simulink model "hyd_hyb_2_int_cont_Final_AMT"  (R2013b)
settings: Solver=ode4  StartTime=0  StopTime=3005  FixedStep=0.01  MaxStep=.4  RelTol=1e-8
InitFcn:
  | const_3_new
values from neighbouring files (symbols this model uses):
  Af = 6.3    [brk_enrg.m]    (also in brk_enrg_1.m)
  BSFC_906_205 = [3.5684 4.3466 5.1668 6.0769 6.988 7.8992 8.8104 9.7336 10.8548 11.9809 13.1112 14.2571 ... (663 elements, 39x17)]    [BSFC_map_906_205.mat]
  Cd = 0.55    [brk_enrg.m]    (also in brk_enrg_1.m)
  den = 1.202    [brk_enrg.m]    (also in brk_enrg_1.m)
  fr = 0.01    [brk_enrg.m]    (also in brk_enrg_1.m)
undefined symbols (not defined in the file or in its folder): clutchRise, down_spd_2, down_spd_3, down_spd_4, down_spd_c, Driving_Cycle, fuel_density, gearshift, I_wheel, Idle_spd_eng_906, M1_hydr, p_v_15, pmax_125, qv_125, Rw, sec_eng_sfc_map, T0, T1, T_max_906, T_min, TC_spd_ratio_max, teta_new_10, torque_convertor, Twait, up_spd_1, up_spd_2, up_spd_3, up_spd_c, v_p_10, v_p_15, v_p_5
libraries: neural x1742, fl_lib x43, nesl_utility x30, sdl_lib x14, simulink x4, simulink_need_slupdate x1
(part 18 of 26)

== system hyd_hyb_2_int_cont_Final_AMT/controller1/optimized controller/SOC upper 0.5/SOC upper 0.6/SOC under 0.7/net_loc_rod_6_7/Layer 3/Delays 1 ==
  "p{3}" : Inport  PortDimensions=65
  mux : Mux  Inputs=1
  "pd{3,2}" : Outport
  wires:
  mux/1 -> "pd{3,2}"/1
  "p{3}"/1 -> mux/1

== system hyd_hyb_2_int_cont_Final_AMT/controller1/optimized controller/SOC upper 0.5/SOC upper 0.6/SOC under 0.7/net_loc_rod_6_7/Layer 3/LW{3,2} ==
  "ad{3,2}" : Inport  PortDimensions=65
  "IW{3,2}(1,:)'" : Constant  Value=[-0.21190558148273514;-0.028250456332647261;0.33957139945877679;0.19274652478953275;-0.42961698454965908;0.23052255270038227;-0.37497561736022994;-0.06185645589928139;0.01165116263494341;-0.15963912751743919;-0.87324175537425064;0.10590816804656823;0.069053323215663556;0.077910861425516578;-0.16798922620742043;-0.22056720645742031;0.13367494956427081;0.36136249854843466;-0.50239119110845365;0.012331807086952057;-0.096965686807043844;0.11986982112408856;-0.31830050450261449;0.11706810526331732;-0.52980599528072625;-0.29641942316489694;0.17415062016965829;-0.098905843864114676;-0.27508713459790696;-0.033419612327731621;-0.2254339214197735;0.027831220456353004;0.29925289926941745;-0.070435212430303012;0.29619502791901131;-0.47601606724683371;-0.22767027734105019;0.41339738030579964;-0.26217552491145868;-0.036734014287553567;-0.55981845033730226;-0.83512658858317002;-0.056808057570803309;-0.22345195834484222;-0.28036785465301478;-0.22949243361228511;-0.34209162741874338;-0.39092697900045326;0.32531105678992528;0.10423076111174255;0.2359871210092597;-0.47216686128522006;-0.20439924920680128;-0.11922663531256097;-0.019922601561886109;0.044510324605291363;-0.27729290371229609;-0.36614438332522081;0.816368987577891;0.54191447654746938;0.5157713773005137;0.26230341773617905;0.70532547287095315;0.23331847514630705;-0.046156806107243299]
  Mux : Mux  Inputs=1
  dotprod1 : neural/Weight Functions/dotprod
  "lz{3,2}" : Outport
  wires:
  Mux/1 -> "lz{3,2}"/1
  dotprod1/1 -> Mux/1
  "ad{3,2}"/1 -> dotprod1/2
  "IW{3,2}(1,:)'"/1 -> dotprod1/1

== system hyd_hyb_2_int_cont_Final_AMT/controller1/optimized controller/SOC upper 0.5/SOC upper 0.6/SOC upper 0.7/SOC under 0.8/net_col_a_b_7_8/Layer 1 ==
  "p{1}" : Inport  PortDimensions=2
  Delays 1 : Subsystem
  "IW{1,1}" : Subsystem
  "b{1}" : Constant  Value=[8.2916467646585872;-7.8114778185757023;-7.3358740319827671;-6.8287428687854348;6.3257902864971145;5.7992770695782818;5.3094756346830199;4.9115066356687667;-4.3713108462153514;-3.8883509962050646;3.3793456803311566;2.8729633399532961;-2.4756245359899856;1.6763370386535841;1.5305900525159519;0.90882364470135646;0.44992343591511891;0.040547487289665569;0.62387277578531353;-1.1506418258106572;1.8779212144940651;1.9372314274500504;2.3477899083139837;2.9384613260166579;-3.1569713919719704;3.945195331065702;-4.46999394454709;-4.8935944330051546;5.3383406441107919;-5.8921601467554003;-6.437017113135763;-6.6308369147221251;-7.2519979683223239;7.7912717207669244;-8.2765880656885411]
  netsum : Sum  Inputs=2  SaturateOnIntegerOverflow=on  InputSameDT=on  OutDataTypeStr=Inherit: Same as first input
  tansig : neural/Transfer Functions/tansig
  "a{1}" : Outport  InitialOutput=[0;0;0;0;0;0;0;0;0;0;0;0;0;0;0;0;0;0;0;0;0;0;0;0;0;0;0;0;0;0;0;0;0;0;0]
  wires:
  tansig/1 -> "a{1}"/1
  netsum/1 -> tansig/1
  "b{1}"/1 -> netsum/2
  "IW{1,1}"/1("iz{1,1}") -> netsum/1
  Delays 1/1("pd{1,1}") -> "IW{1,1}"/1("pd{1,1}")
  "p{1}"/1 -> Delays 1/1("p{1}")

== system hyd_hyb_2_int_cont_Final_AMT/controller1/optimized controller/SOC upper 0.5/SOC upper 0.6/SOC upper 0.7/SOC under 0.8/net_col_a_b_7_8/Layer 2 ==
  "a{1} " : Inport  PortDimensions=35
  Delays 1 : Subsystem
  "LW{2,1}" : Subsystem
  "b{2}" : Constant  Value=[1.6246025903810972;-1.5137529513143568;1.4133649641113548;1.3507873768326613;1.2831264026044094;-1.1583875849183927;-1.1687705629463485;-1.0638601573162123;-0.97507485546902606;-0.92163063226781328;-0.85414749875120755;-0.81745251898413263;0.71780688605314269;0.64596911275152968;-0.5713050323286234;0.44864531658767243;-0.44458366605836119;-0.39178178454963697;-0.30831552725782874;-0.2030923610966566;-0.17177709670230834;-0.089970322460785082;0.045878470178160817;0.077082912036474494;-0.18386481774142041;0.2395566239489996;0.27679632832356704;0.35435254107540132;0.43035932518500436;-0.49005207867104572;-0.61109910818045332;-0.69212605142728045;-0.70628312057121345;0.72592925676845665;-0.82226073192444138;-0.92563474243113997;0.91244556659384735;1.0573029525194646;1.1239522443373839;1.2068081707832854;1.2709694444207866;1.357007844557339;-1.4138174953273674;1.4928009886700373;1.5432286468653338]
  netsum : Sum  Inputs=2  SaturateOnIntegerOverflow=on  InputSameDT=on  OutDataTypeStr=Inherit: Same as first input
  tansig : neural/Transfer Functions/tansig
  "a{2}" : Outport  InitialOutput=[0;0;0;0;0;0;0;0;0;0;0;0;0;0;0;0;0;0;0;0;0;0;0;0;0;0;0;0;0;0;0;0;0;0;0;0;0;0;0;0;0;0;0;0;0]
  wires:
  tansig/1 -> "a{2}"/1
  netsum/1 -> tansig/1
  "b{2}"/1 -> netsum/2
  "LW{2,1}"/1("lz{2,1}") -> netsum/1
  Delays 1/1("pd{2,1}") -> "LW{2,1}"/1("ad{2,1}")
  "a{1} "/1 -> Delays 1/1("p{2}")

== system hyd_hyb_2_int_cont_Final_AMT/controller1/optimized controller/SOC upper 0.5/SOC upper 0.6/SOC upper 0.7/SOC under 0.8/net_col_a_b_7_8/Layer 3 ==
  "a{2} " : Inport  PortDimensions=45
  Delays 1 : Subsystem
  "LW{3,2}" : Subsystem
  "b{3}" : Constant  Value=0.43583087047788488
  netsum : Sum  Inputs=2  SaturateOnIntegerOverflow=on  InputSameDT=on  OutDataTypeStr=Inherit: Same as first input
  purelin : neural/Transfer Functions/purelin
  "a{3}" : Outport  InitialOutput=0
  wires:
  purelin/1 -> "a{3}"/1
  netsum/1 -> purelin/1
  "b{3}"/1 -> netsum/2
  "LW{3,2}"/1("lz{3,2}") -> netsum/1
  Delays 1/1("pd{3,2}") -> "LW{3,2}"/1("ad{3,2}")
  "a{2} "/1 -> Delays 1/1("p{3}")

== system hyd_hyb_2_int_cont_Final_AMT/controller1/optimized controller/SOC upper 0.5/SOC upper 0.6/SOC upper 0.7/SOC under 0.8/net_col_a_b_7_8/Process Input 1 ==
  x : Inport  PortDimensions=2
  fixunknowns : neural/Processing Functions/fixunknowns  inputSize=2  indices=[1 2]
  mapminmax : neural/Processing Functions/mapminmax  xmin=[0.0050576114402896234;0.2341095]  xmax=[1;0.94609200000000004]  ymin=-1  ymax=1
  removeconstantrows : neural/Processing Functions/removeconstantrows  inputSize=2  keep=[1 2]
  p : Outport  PortDimensions=2
  wires:
  mapminmax/1 -> p/1
  removeconstantrows/1 -> mapminmax/1
  fixunknowns/1 -> removeconstantrows/1
  x/1 -> fixunknowns/1

== system hyd_hyb_2_int_cont_Final_AMT/controller1/optimized controller/SOC upper 0.5/SOC upper 0.6/SOC upper 0.7/SOC under 0.8/net_col_a_b_7_8/Process Output 1 ==
  a : Inport  PortDimensions=1
  mapminmax_reverse : neural/Processing Functions/mapminmax_reverse  xmin=0  xmax=1  ymin=-1  ymax=1
  removeconstantrows_reverse : neural/Processing Functions/removeconstantrows_reverse  inputSize=1  constants=zeros(0,1)  rearrange=1
  y : Outport  PortDimensions=1
  wires:
  removeconstantrows_reverse/1 -> y/1
  mapminmax_reverse/1 -> removeconstantrows_reverse/1
  a/1 -> mapminmax_reverse/1

== system hyd_hyb_2_int_cont_Final_AMT/controller1/optimized controller/SOC upper 0.5/SOC upper 0.6/SOC upper 0.7/SOC under 0.8/net_col_c_d_7_8/Layer 1 ==
  "p{1}" : Inport  PortDimensions=2
  Delays 1 : Subsystem
  "IW{1,1}" : Subsystem
  "b{1}" : Constant  Value=[8.3116902859191448;7.8029060171194731;7.2867035561831317;6.8260213470550735;6.346607988807234;5.8562497365900965;-5.3743261762591725;4.9530955883541345;-4.383911258273109;-3.8970793742576069;-3.4314686513161763;2.863791263998738;2.4209773053043331;1.956446882392439;-1.4732357207624023;-0.86517942611961574;-0.48032492618428974;-0.026719041791466704;0.45434793064694279;0.96417086831869769;-1.4746840868110174;-1.932288244085119;-2.4708323565900367;-2.9643399257520366;-3.430878366683491;3.8862801103928728;4.3962114473631928;4.8870263091686326;-5.3420629575502314;-5.8367411293877227;-6.4407592729025556;6.809228192120738;7.3082174034078067;7.795329331848893;8.3148626555089304]
  netsum : Sum  Inputs=2  SaturateOnIntegerOverflow=on  InputSameDT=on  OutDataTypeStr=Inherit: Same as first input
  tansig : neural/Transfer Functions/tansig
  "a{1}" : Outport  InitialOutput=[0;0;0;0;0;0;0;0;0;0;0;0;0;0;0;0;0;0;0;0;0;0;0;0;0;0;0;0;0;0;0;0;0;0;0]
  wires:
  tansig/1 -> "a{1}"/1
  netsum/1 -> tansig/1
  "b{1}"/1 -> netsum/2
  "IW{1,1}"/1("iz{1,1}") -> netsum/1
  Delays 1/1("pd{1,1}") -> "IW{1,1}"/1("pd{1,1}")
  "p{1}"/1 -> Delays 1/1("p{1}")

== system hyd_hyb_2_int_cont_Final_AMT/controller1/optimized controller/SOC upper 0.5/SOC upper 0.6/SOC upper 0.7/SOC under 0.8/net_col_c_d_7_8/Layer 2 ==
  "a{1} " : Inport  PortDimensions=35
  Delays 1 : Subsystem
  "LW{2,1}" : Subsystem
  "b{2}" : Constant  Value=[-1.5686018942941038;-1.4913194182180465;1.4364195261274875;1.3923653246708561;-1.3174444073080744;-1.2329202605406324;-1.2231091177906401;-1.1113434209070936;1.0523981087233136;-1.0082372091808669;-0.93678500720920321;-0.85933642747852601;0.79256290609693925;0.7194191061208759;0.62735773675601636;-0.63057612726771706;0.52881759345176838;0.4726739238819378;-0.36991235182195747;0.39954692502574662;0.32402525688235295;-0.25368530430266362;-0.16353113859080878;0.1147228728047736;-0.058400493998987592;0.033005568957060874;-0.052329484615956483;-0.10924330494808851;-0.19798005180984199;-0.29896342389825387;0.35766529096251598;0.42867990671694767;0.4489209967696316;0.53972993122561663;0.6167646902802062;-0.61139064819023359;-0.74306982939588972;-0.76508190452300739;-0.87147423129092416;0.94153999709968716;-0.99016236737475172;-1.0232275653663527;-1.1417743437718129;1.1612439923201026;-1.1779260494401698;1.2812899302236036;1.3707661966465723;1.4742421981136882;-1.47793500374455;-1.5586030678282377]
  netsum : Sum  Inputs=2  SaturateOnIntegerOverflow=on  InputSameDT=on  OutDataTypeStr=Inherit: Same as first input
  tansig : neural/Transfer Functions/tansig
  "a{2}" : Outport  InitialOutput=[0;0;0;0;0;0;0;0;0;0;0;0;0;0;0;0;0;0;0;0;0;0;0;0;0;0;0;0;0;0;0;0;0;0;0;0;0;0;0;0;0;0;0;0;0;0;0;0;0;0]
  wires:
  tansig/1 -> "a{2}"/1
  netsum/1 -> tansig/1
  "b{2}"/1 -> netsum/2
  "LW{2,1}"/1("lz{2,1}") -> netsum/1
  Delays 1/1("pd{2,1}") -> "LW{2,1}"/1("ad{2,1}")
  "a{1} "/1 -> Delays 1/1("p{2}")

== system hyd_hyb_2_int_cont_Final_AMT/controller1/optimized controller/SOC upper 0.5/SOC upper 0.6/SOC upper 0.7/SOC under 0.8/net_col_c_d_7_8/Layer 3 ==
  "a{2} " : Inport  PortDimensions=50
  Delays 1 : Subsystem
  "LW{3,2}" : Subsystem
  "b{3}" : Constant  Value=-0.33436314693187646
  netsum : Sum  Inputs=2  SaturateOnIntegerOverflow=on  InputSameDT=on  OutDataTypeStr=Inherit: Same as first input
  purelin : neural/Transfer Functions/purelin
  "a{3}" : Outport  InitialOutput=0
  wires:
  purelin/1 -> "a{3}"/1
  netsum/1 -> purelin/1
  "b{3}"/1 -> netsum/2
  "LW{3,2}"/1("lz{3,2}") -> netsum/1
  Delays 1/1("pd{3,2}") -> "LW{3,2}"/1("ad{3,2}")
  "a{2} "/1 -> Delays 1/1("p{3}")

== system hyd_hyb_2_int_cont_Final_AMT/controller1/optimized controller/SOC upper 0.5/SOC upper 0.6/SOC upper 0.7/SOC under 0.8/net_col_c_d_7_8/Process Input 1 ==
  x : Inport  PortDimensions=2
  fixunknowns : neural/Processing Functions/fixunknowns  inputSize=2  indices=[1 2]
  mapminmax : neural/Processing Functions/mapminmax  xmin=[0.11115622208057092;0.17457650000000002]  xmax=[1;0.653254]  ymin=-1  ymax=1
  removeconstantrows : neural/Processing Functions/removeconstantrows  inputSize=2  keep=[1 2]
  p : Outport  PortDimensions=2
  wires:
  mapminmax/1 -> p/1
  removeconstantrows/1 -> mapminmax/1
  fixunknowns/1 -> removeconstantrows/1
  x/1 -> fixunknowns/1

== system hyd_hyb_2_int_cont_Final_AMT/controller1/optimized controller/SOC upper 0.5/SOC upper 0.6/SOC upper 0.7/SOC under 0.8/net_col_c_d_7_8/Process Output 1 ==
  a : Inport  PortDimensions=1
  mapminmax_reverse : neural/Processing Functions/mapminmax_reverse  xmin=0  xmax=1  ymin=-1  ymax=1
  removeconstantrows_reverse : neural/Processing Functions/removeconstantrows_reverse  inputSize=1  constants=zeros(0,1)  rearrange=1
  y : Outport  PortDimensions=1
  wires:
  removeconstantrows_reverse/1 -> y/1
  mapminmax_reverse/1 -> removeconstantrows_reverse/1
  a/1 -> mapminmax_reverse/1

== system hyd_hyb_2_int_cont_Final_AMT/controller1/optimized controller/SOC upper 0.5/SOC upper 0.6/SOC upper 0.7/SOC under 0.8/net_col_e_f_7_8/Layer 1 ==
  "p{1}" : Inport  PortDimensions=2
  Delays 1 : Subsystem
  "IW{1,1}" : Subsystem
  "b{1}" : Constant  Value=[-7.6881018002993811;-7.1696124955463407;6.6274067676391244;-6.1028538948157074;-5.5114890432277486;5.0228105143392874;-4.3713949897040196;-3.9579533195973844;-3.5424320446653481;-2.9063109252236838;2.3884921851729382;-1.8701611263712352;-1.3278082575057837;-0.7034153508496056;-0.29496096693313423;-0.24905479630949848;0.64349556452967571;-1.3288485356492385;-1.8412347415254877;2.3729253819088352;2.9176813905058485;-3.4852070547888778;-3.9696003266601889;-4.4547493683646611;-5.0158733055263856;5.560382862684909;6.0845307363798815;-6.6092525461039449;7.1485320918848041;7.6474074439409838]
  netsum : Sum  Inputs=2  SaturateOnIntegerOverflow=on  InputSameDT=on  OutDataTypeStr=Inherit: Same as first input
  tansig : neural/Transfer Functions/tansig
  "a{1}" : Outport  InitialOutput=[0;0;0;0;0;0;0;0;0;0;0;0;0;0;0;0;0;0;0;0;0;0;0;0;0;0;0;0;0;0]
  wires:
  tansig/1 -> "a{1}"/1
  netsum/1 -> tansig/1
  "b{1}"/1 -> netsum/2
  "IW{1,1}"/1("iz{1,1}") -> netsum/1
  Delays 1/1("pd{1,1}") -> "IW{1,1}"/1("pd{1,1}")
  "p{1}"/1 -> Delays 1/1("p{1}")

== system hyd_hyb_2_int_cont_Final_AMT/controller1/optimized controller/SOC upper 0.5/SOC upper 0.6/SOC upper 0.7/SOC under 0.8/net_col_e_f_7_8/Layer 2 ==
  "a{1} " : Inport  PortDimensions=30
  Delays 1 : Subsystem
  "LW{2,1}" : Subsystem
  "b{2}" : Constant  Value=[-1.5477297612963636;-1.5293021250108161;-1.4865534978599506;-1.4350225305745659;-1.3320349172545887;1.2759493127119488;1.2067092228755465;1.1585040165641989;1.0818111732552;-1.0217707490071199;-0.93625284533737974;0.86084334590742473;-0.81611566901033294;-0.75977572837522622;-0.68195671405109437;0.61250166315132237;0.56784720520380716;-0.47392917471101453;-0.42294051348806871;-0.34059086854467668;0.28432035961595142;-0.26239849492555123;0.16655305034653378;0.09689078681840467;-0.043301963584861977;0.032103319387171828;0.13394593375940797;0.18086752211467982;-0.1880786349548369;-0.29610569226816436;0.35856623667981335;-0.44696828544509076;0.48850426202371683;-0.4992446928319636;0.60332468246739523;-0.68407090563130457;0.75073264123508454;0.83254585737929787;0.85952336377303395;-0.95829921584290212;1.0048957119927975;1.0901091238963656;-1.1625782212970923;1.206521081803045;1.2660766711955194;-1.3373607373409551;-1.4184409448334543;1.4527994853647119;1.5068978308092387;1.6095996810907955]
  netsum : Sum  Inputs=2  SaturateOnIntegerOverflow=on  InputSameDT=on  OutDataTypeStr=Inherit: Same as first input
  tansig : neural/Transfer Functions/tansig
  "a{2}" : Outport  InitialOutput=[0;0;0;0;0;0;0;0;0;0;0;0;0;0;0;0;0;0;0;0;0;0;0;0;0;0;0;0;0;0;0;0;0;0;0;0;0;0;0;0;0;0;0;0;0;0;0;0;0;0]
  wires:
  tansig/1 -> "a{2}"/1
  netsum/1 -> tansig/1
  "b{2}"/1 -> netsum/2
  "LW{2,1}"/1("lz{2,1}") -> netsum/1
  Delays 1/1("pd{2,1}") -> "LW{2,1}"/1("ad{2,1}")
  "a{1} "/1 -> Delays 1/1("p{2}")

== system hyd_hyb_2_int_cont_Final_AMT/controller1/optimized controller/SOC upper 0.5/SOC upper 0.6/SOC upper 0.7/SOC under 0.8/net_col_e_f_7_8/Layer 3 ==
  "a{2} " : Inport  PortDimensions=50
  Delays 1 : Subsystem
  "LW{3,2}" : Subsystem
  "b{3}" : Constant  Value=-0.46106071391077463
  netsum : Sum  Inputs=2  SaturateOnIntegerOverflow=on  InputSameDT=on  OutDataTypeStr=Inherit: Same as first input
  purelin : neural/Transfer Functions/purelin
  "a{3}" : Outport  InitialOutput=0
  wires:
  purelin/1 -> "a{3}"/1
  netsum/1 -> purelin/1
  "b{3}"/1 -> netsum/2
  "LW{3,2}"/1("lz{3,2}") -> netsum/1
  Delays 1/1("pd{3,2}") -> "LW{3,2}"/1("ad{3,2}")
  "a{2} "/1 -> Delays 1/1("p{3}")

== system hyd_hyb_2_int_cont_Final_AMT/controller1/optimized controller/SOC upper 0.5/SOC upper 0.6/SOC upper 0.7/SOC under 0.8/net_col_e_f_7_8/Process Input 1 ==
  x : Inport  PortDimensions=2
  fixunknowns : neural/Processing Functions/fixunknowns  inputSize=2  indices=[1 2]
  mapminmax : neural/Processing Functions/mapminmax  xmin=[0.00010433375339546994;0.0080852249999999997]  xmax=[1.009090909090909;0.64359999999999995]  ymin=-1  ymax=1
  removeconstantrows : neural/Processing Functions/removeconstantrows  inputSize=2  keep=[1 2]
  p : Outport  PortDimensions=2
  wires:
  mapminmax/1 -> p/1
  removeconstantrows/1 -> mapminmax/1
  fixunknowns/1 -> removeconstantrows/1
  x/1 -> fixunknowns/1

== system hyd_hyb_2_int_cont_Final_AMT/controller1/optimized controller/SOC upper 0.5/SOC upper 0.6/SOC upper 0.7/SOC under 0.8/net_col_e_f_7_8/Process Output 1 ==
  a : Inport  PortDimensions=1
  mapminmax_reverse : neural/Processing Functions/mapminmax_reverse  xmin=0  xmax=1  ymin=-1  ymax=1
  removeconstantrows_reverse : neural/Processing Functions/removeconstantrows_reverse  inputSize=1  constants=zeros(0,1)  rearrange=1
  y : Outport  PortDimensions=1
  wires:
  removeconstantrows_reverse/1 -> y/1
  mapminmax_reverse/1 -> removeconstantrows_reverse/1
  a/1 -> mapminmax_reverse/1

== system hyd_hyb_2_int_cont_Final_AMT/controller1/optimized controller/SOC upper 0.5/SOC upper 0.6/SOC upper 0.7/SOC under 0.8/net_loc_rod_7_8/Layer 1 ==
  "p{1}" : Inport  PortDimensions=2
  Delays 1 : Subsystem
  "IW{1,1}" : Subsystem
  "b{1}" : Constant  Value=[-7.6664348708937533;7.1445971682878477;6.6167168492832911;6.0860061370357288;-5.5315107878025573;5.0261307682562233;-4.494082622797607;4.0719078555663542;3.4709759431734448;2.9188468639647454;2.3943935266761707;1.8335702310625019;1.3202491244505703;-0.76888435535120259;0.24778438862887789;0.33462371266191271;-0.76243416083955973;1.3762346449687806;1.9102702785135495;-2.3929428850095324;-2.9022803344286112;-3.690412197637341;3.9573609372276932;-4.5993292631946163;-5.0475261103641618;5.4709604300797592;6.077408482873671;6.5770239742392009;7.1375905348778197;7.6179993162728579]
  netsum : Sum  Inputs=2  SaturateOnIntegerOverflow=on  InputSameDT=on  OutDataTypeStr=Inherit: Same as first input
  tansig : neural/Transfer Functions/tansig
  "a{1}" : Outport  InitialOutput=[0;0;0;0;0;0;0;0;0;0;0;0;0;0;0;0;0;0;0;0;0;0;0;0;0;0;0;0;0;0]
  wires:
  tansig/1 -> "a{1}"/1
  netsum/1 -> tansig/1
  "b{1}"/1 -> netsum/2
  "IW{1,1}"/1("iz{1,1}") -> netsum/1
  Delays 1/1("pd{1,1}") -> "IW{1,1}"/1("pd{1,1}")
  "p{1}"/1 -> Delays 1/1("p{1}")

== system hyd_hyb_2_int_cont_Final_AMT/controller1/optimized controller/SOC upper 0.5/SOC upper 0.6/SOC upper 0.7/SOC under 0.8/net_loc_rod_7_8/Layer 2 ==
  "a{1} " : Inport  PortDimensions=30
  Delays 1 : Subsystem
  "LW{2,1}" : Subsystem
  "b{2}" : Constant  Value=[1.5809057638664712;1.5807151854123314;1.4855560118917412;1.4342816648463235;-1.3852838862690111;-1.3763643250737478;-1.2699307671350113;1.2284424739443496;-1.1667825506616738;1.1126454079697519;1.0473054037992569;0.99287875006871451;-0.95329260687326012;0.83638794087360679;-0.83792818135557123;-0.78046148241162161;-0.71425010683179146;0.68949490542424974;0.64329890641382304;0.57899988405152292;-0.47143091913162039;-0.47926974452184956;-0.40398687055644222;-0.35659194048479592;0.30321322377409698;-0.27451350524017853;-0.1767238128948169;0.16987849996636148;0.080295435290659523;-0.029950542574714353;0.027089350482413167;0.058629507356316252;0.15615280386139965;-0.20370835576685978;0.24221681438327167;0.28202876584714487;-0.38246747542268622;0.41676300939491745;-0.45528940316231631;0.52075351132689529;-0.571489263720799;0.64385068877791618;-0.69328786198464676;0.7382904151092311;-0.7686738347751072;0.84397313956728726;-0.88866651589897194;0.96837105796755452;1.0162563106498559;-1.0533618556353999;-1.0943063056832119;-1.1877806527843298;-1.2159917192725045;-1.253506527704173;1.3326748437569171;1.3938223174811426;1.4658688434887885;1.4916223339098742;1.5398710502961235;1.601176272795612]
  netsum : Sum  Inputs=2  SaturateOnIntegerOverflow=on  InputSameDT=on  OutDataTypeStr=Inherit: Same as first input
  tansig : neural/Transfer Functions/tansig
  "a{2}" : Outport  InitialOutput=[0;0;0;0;0;0;0;0;0;0;0;0;0;0;0;0;0;0;0;0;0;0;0;0;0;0;0;0;0;0;0;0;0;0;0;0;0;0;0;0;0;0;0;0;0;0;0;0;0;0;0;0;0;0;0;0;0;0;0;0]
  wires:
  tansig/1 -> "a{2}"/1
  netsum/1 -> tansig/1
  "b{2}"/1 -> netsum/2
  "LW{2,1}"/1("lz{2,1}") -> netsum/1
  Delays 1/1("pd{2,1}") -> "LW{2,1}"/1("ad{2,1}")
  "a{1} "/1 -> Delays 1/1("p{2}")

== system hyd_hyb_2_int_cont_Final_AMT/controller1/optimized controller/SOC upper 0.5/SOC upper 0.6/SOC upper 0.7/SOC under 0.8/net_loc_rod_7_8/Layer 3 ==
  "a{2} " : Inport  PortDimensions=60
  Delays 1 : Subsystem
  "LW{3,2}" : Subsystem
  "b{3}" : Constant  Value=-0.93224771825496566
  netsum : Sum  Inputs=2  SaturateOnIntegerOverflow=on  InputSameDT=on  OutDataTypeStr=Inherit: Same as first input
  purelin : neural/Transfer Functions/purelin
  "a{3}" : Outport  InitialOutput=0
  wires:
  purelin/1 -> "a{3}"/1
  netsum/1 -> purelin/1
  "b{3}"/1 -> netsum/2
  "LW{3,2}"/1("lz{3,2}") -> netsum/1
  Delays 1/1("pd{3,2}") -> "LW{3,2}"/1("ad{3,2}")
  "a{2} "/1 -> Delays 1/1("p{3}")

== system hyd_hyb_2_int_cont_Final_AMT/controller1/optimized controller/SOC upper 0.5/SOC upper 0.6/SOC upper 0.7/SOC under 0.8/net_loc_rod_7_8/Process Input 1 ==
  x : Inport  PortDimensions=2
  fixunknowns : neural/Processing Functions/fixunknowns  inputSize=2  indices=[1 2]
  mapminmax : neural/Processing Functions/mapminmax  xmin=[0.088429741348767466;0.013660410000000001]  xmax=[1;0.49235399999999996]  ymin=-1  ymax=1
  removeconstantrows : neural/Processing Functions/removeconstantrows  inputSize=2  keep=[1 2]
  p : Outport  PortDimensions=2
  wires:
  mapminmax/1 -> p/1
  removeconstantrows/1 -> mapminmax/1
  fixunknowns/1 -> removeconstantrows/1
  x/1 -> fixunknowns/1

== system hyd_hyb_2_int_cont_Final_AMT/controller1/optimized controller/SOC upper 0.5/SOC upper 0.6/SOC upper 0.7/SOC under 0.8/net_loc_rod_7_8/Process Output 1 ==
  a : Inport  PortDimensions=1
  mapminmax_reverse : neural/Processing Functions/mapminmax_reverse  xmin=0  xmax=1  ymin=-1  ymax=1
  removeconstantrows_reverse : neural/Processing Functions/removeconstantrows_reverse  inputSize=1  constants=zeros(0,1)  rearrange=1
  y : Outport  PortDimensions=1
  wires:
  removeconstantrows_reverse/1 -> y/1
  mapminmax_reverse/1 -> removeconstantrows_reverse/1
  a/1 -> mapminmax_reverse/1

== system hyd_hyb_2_int_cont_Final_AMT/controller1/optimized controller/SOC upper 0.5/SOC upper 0.6/SOC upper 0.7/SOC upper 0.8/net_col_a_b_8_9/Layer 1 ==
  "p{1}" : Inport  PortDimensions=2
  Delays 1 : Subsystem
  "IW{1,1}" : Subsystem
  "b{1}" : Constant  Value=[8.2903358215080676;-7.7657998848495637;7.3258361320457999;6.8322940827755767;6.3907366524362228;5.8513299473215454;5.428748873413956;4.8908030844795327;4.4622980602266207;3.9184323697946635;3.4421533237276636;-2.8848117854051845;-2.3908374697190853;1.9426308888625365;-1.4634502352179708;1.0159704232714091;-0.47136167422531949;-0.025928304818340971;0.48223344450605304;0.95348009234162501;1.5262155812589833;-1.9494027462808818;-2.378648219600497;-2.9433743702973341;3.2998478685400348;-3.8872063221167878;4.433440918095731;-4.8693917332986398;5.3487774127091638;5.8086420838160704;-6.3275200720026099;-6.8387453294921219;7.3072846143090002;7.798095465885619;8.2978794542543266]
  netsum : Sum  Inputs=2  SaturateOnIntegerOverflow=on  InputSameDT=on  OutDataTypeStr=Inherit: Same as first input
  tansig : neural/Transfer Functions/tansig
  "a{1}" : Outport  InitialOutput=[0;0;0;0;0;0;0;0;0;0;0;0;0;0;0;0;0;0;0;0;0;0;0;0;0;0;0;0;0;0;0;0;0;0;0]
  wires:
  tansig/1 -> "a{1}"/1
  netsum/1 -> tansig/1
  "b{1}"/1 -> netsum/2
  "IW{1,1}"/1("iz{1,1}") -> netsum/1
  Delays 1/1("pd{1,1}") -> "IW{1,1}"/1("pd{1,1}")
  "p{1}"/1 -> Delays 1/1("p{1}")

== system hyd_hyb_2_int_cont_Final_AMT/controller1/optimized controller/SOC upper 0.5/SOC upper 0.6/SOC upper 0.7/SOC upper 0.8/net_col_a_b_8_9/Layer 2 ==
  "a{1} " : Inport  PortDimensions=35
  Delays 1 : Subsystem
  "LW{2,1}" : Subsystem
  "b{2}" : Constant  Value=[1.5516475171408779;1.4835098818771537;1.4312277511141751;-1.3698842963986313;-1.2806997344309183;-1.1693837969306802;-1.1407058875630671;-1.0781990386589757;-1.0357595176145418;0.90372054013783332;0.85261985678638907;0.76193934695339194;0.75173184958776618;0.66413214424768063;0.5671249522564511;0.51661208652598578;0.40848110978741226;0.36021562083255332;-0.28984413185003965;-0.21008240837066611;-0.10811356805866763;0.078212987099658043;0.050261178409190178;-0.062855911586719854;-0.15960669841975192;-0.29221472137958321;0.30888189547496875;-0.37759084863654085;0.39785437443106902;0.5025042997703113;0.6852123648390992;0.57126476826852779;-0.72454872028325679;-0.81256808327758079;0.92122536494791152;-0.94207467763840702;1.0352444398307015;1.0564038748070703;1.1414641552110378;1.1803996896086595;-1.3183578069980528;-1.3096087100254543;1.3521491510226666;1.5210842316929682;1.5661396273710371]
  netsum : Sum  Inputs=2  SaturateOnIntegerOverflow=on  InputSameDT=on  OutDataTypeStr=Inherit: Same as first input
  tansig : neural/Transfer Functions/tansig
  "a{2}" : Outport  InitialOutput=[0;0;0;0;0;0;0;0;0;0;0;0;0;0;0;0;0;0;0;0;0;0;0;0;0;0;0;0;0;0;0;0;0;0;0;0;0;0;0;0;0;0;0;0;0]
  wires:
  tansig/1 -> "a{2}"/1
  netsum/1 -> tansig/1
  "b{2}"/1 -> netsum/2
  "LW{2,1}"/1("lz{2,1}") -> netsum/1
  Delays 1/1("pd{2,1}") -> "LW{2,1}"/1("ad{2,1}")
  "a{1} "/1 -> Delays 1/1("p{2}")

== system hyd_hyb_2_int_cont_Final_AMT/controller1/optimized controller/SOC upper 0.5/SOC upper 0.6/SOC upper 0.7/SOC upper 0.8/net_col_a_b_8_9/Layer 3 ==
  "a{2} " : Inport  PortDimensions=45
  Delays 1 : Subsystem
  "LW{3,2}" : Subsystem
  "b{3}" : Constant  Value=0.6155887857634984
  netsum : Sum  Inputs=2  SaturateOnIntegerOverflow=on  InputSameDT=on  OutDataTypeStr=Inherit: Same as first input
  purelin : neural/Transfer Functions/purelin
  "a{3}" : Outport  InitialOutput=0
  wires:
  purelin/1 -> "a{3}"/1
  netsum/1 -> purelin/1
  "b{3}"/1 -> netsum/2
  "LW{3,2}"/1("lz{3,2}") -> netsum/1
  Delays 1/1("pd{3,2}") -> "LW{3,2}"/1("ad{3,2}")
  "a{2} "/1 -> Delays 1/1("p{3}")

== system hyd_hyb_2_int_cont_Final_AMT/controller1/optimized controller/SOC upper 0.5/SOC upper 0.6/SOC upper 0.7/SOC upper 0.8/net_col_a_b_8_9/Process Input 1 ==
  x : Inport  PortDimensions=2
  fixunknowns : neural/Processing Functions/fixunknowns  inputSize=2  indices=[1 2]
  mapminmax : neural/Processing Functions/mapminmax  xmin=[0.0003822621604903857;0.041431750000000003]  xmax=[1;0.69701880000000005]  ymin=-1  ymax=1
  removeconstantrows : neural/Processing Functions/removeconstantrows  inputSize=2  keep=[1 2]
  p : Outport  PortDimensions=2
  wires:
  mapminmax/1 -> p/1
  removeconstantrows/1 -> mapminmax/1
  fixunknowns/1 -> removeconstantrows/1
  x/1 -> fixunknowns/1

== system hyd_hyb_2_int_cont_Final_AMT/controller1/optimized controller/SOC upper 0.5/SOC upper 0.6/SOC upper 0.7/SOC upper 0.8/net_col_a_b_8_9/Process Output 1 ==
  a : Inport  PortDimensions=1
  mapminmax_reverse : neural/Processing Functions/mapminmax_reverse  xmin=0  xmax=1  ymin=-1  ymax=1
  removeconstantrows_reverse : neural/Processing Functions/removeconstantrows_reverse  inputSize=1  constants=zeros(0,1)  rearrange=1
  y : Outport  PortDimensions=1
  wires:
  removeconstantrows_reverse/1 -> y/1
  mapminmax_reverse/1 -> removeconstantrows_reverse/1
  a/1 -> mapminmax_reverse/1

== system hyd_hyb_2_int_cont_Final_AMT/controller1/optimized controller/SOC upper 0.5/SOC upper 0.6/SOC upper 0.7/SOC upper 0.8/net_col_c_d_8_9/Layer 1 ==
  "p{1}" : Inport  PortDimensions=2
  Delays 1 : Subsystem
  "IW{1,1}" : Subsystem
  "b{1}" : Constant  Value=[-7.6524589954305595;7.1575966111085725;-6.654801813906313;-6.062921949452706;-5.5671598839301657;-5.0521178951183314;4.5110838179576307;3.946782880463152;3.4022759889300365;-2.9332570607530637;2.3847485055726749;1.930372285371202;-1.4382019821303194;0.77000183863714244;-0.26225474692650153;-0.20738493161860463;0.79875786224452561;1.314952811728606;1.8171463545761435;2.2799587853155048;2.9303600998292048;3.4808110827958494;3.9748206575799894;4.5187216997884914;-5.0721055404459179;5.5382016443803641;6.2740684597329439;6.4514085496008367;-7.3392600553068776;7.5659178060488959]
  netsum : Sum  Inputs=2  SaturateOnIntegerOverflow=on  InputSameDT=on  OutDataTypeStr=Inherit: Same as first input
  tansig : neural/Transfer Functions/tansig
  "a{1}" : Outport  InitialOutput=[0;0;0;0;0;0;0;0;0;0;0;0;0;0;0;0;0;0;0;0;0;0;0;0;0;0;0;0;0;0]
  wires:
  tansig/1 -> "a{1}"/1
  netsum/1 -> tansig/1
  "b{1}"/1 -> netsum/2
  "IW{1,1}"/1("iz{1,1}") -> netsum/1
  Delays 1/1("pd{1,1}") -> "IW{1,1}"/1("pd{1,1}")
  "p{1}"/1 -> Delays 1/1("p{1}")

== system hyd_hyb_2_int_cont_Final_AMT/controller1/optimized controller/SOC upper 0.5/SOC upper 0.6/SOC upper 0.7/SOC upper 0.8/net_col_c_d_8_9/Layer 2 ==
  "a{1} " : Inport  PortDimensions=30
  Delays 1 : Subsystem
  "LW{2,1}" : Subsystem
  "b{2}" : Constant  Value=[-1.5287022483014878;1.5426403940657185;-1.4614221356586912;1.3400868618459401;-1.2027676831476171;-1.2178358987324378;-1.0910327499881933;-1.0404872041228237;-0.9206407025162644;0.82096842682832016;-0.81597475436367373;0.70513330671674967;0.5942273025863497;-0.57573907549896008;-0.36643092989287496;-0.41499221347877618;0.27330592040460605;-0.19900672217238721;0.12188682845735625;0.099377692896292932;-0.048454168804516924;0.11918352171058183;-0.2007677246837809;-0.26479653336079806;-0.34453332666848635;0.42671542704119692;0.5146335294347133;0.62751706753897618;-0.67658170183233923;-0.79975832025806681;-0.86684211752692231;-0.92593317836401323;1.0152616108508217;1.0935118102424268;-1.184870758657562;-1.2348820260904967;1.3200273808778371;1.4157163141339153;-1.4512197794490678;1.574504628514257]
  netsum : Sum  Inputs=2  SaturateOnIntegerOverflow=on  InputSameDT=on  OutDataTypeStr=Inherit: Same as first input
  tansig : neural/Transfer Functions/tansig
  "a{2}" : Outport  InitialOutput=[0;0;0;0;0;0;0;0;0;0;0;0;0;0;0;0;0;0;0;0;0;0;0;0;0;0;0;0;0;0;0;0;0;0;0;0;0;0;0;0]
  wires:
  tansig/1 -> "a{2}"/1
  netsum/1 -> tansig/1
  "b{2}"/1 -> netsum/2
  "LW{2,1}"/1("lz{2,1}") -> netsum/1
  Delays 1/1("pd{2,1}") -> "LW{2,1}"/1("ad{2,1}")
  "a{1} "/1 -> Delays 1/1("p{2}")

== system hyd_hyb_2_int_cont_Final_AMT/controller1/optimized controller/SOC upper 0.5/SOC upper 0.6/SOC upper 0.7/SOC upper 0.8/net_col_c_d_8_9/Layer 3 ==
  "a{2} " : Inport  PortDimensions=40
  Delays 1 : Subsystem
  "LW{3,2}" : Subsystem
  "b{3}" : Constant  Value=0.9979622803312711
  netsum : Sum  Inputs=2  SaturateOnIntegerOverflow=on  InputSameDT=on  OutDataTypeStr=Inherit: Same as first input
  purelin : neural/Transfer Functions/purelin
  "a{3}" : Outport  InitialOutput=0
  wires:
  purelin/1 -> "a{3}"/1
  netsum/1 -> purelin/1
  "b{3}"/1 -> netsum/2
  "LW{3,2}"/1("lz{3,2}") -> netsum/1
  Delays 1/1("pd{3,2}") -> "LW{3,2}"/1("ad{3,2}")
  "a{2} "/1 -> Delays 1/1("p{3}")

== system hyd_hyb_2_int_cont_Final_AMT/controller1/optimized controller/SOC upper 0.5/SOC upper 0.6/SOC upper 0.7/SOC upper 0.8/net_col_c_d_8_9/Process Input 1 ==
  x : Inport  PortDimensions=2
  fixunknowns : neural/Processing Functions/fixunknowns  inputSize=2  indices=[1 2]
  mapminmax : neural/Processing Functions/mapminmax  xmin=[0.0094276106161651479;0.0091891777777777812]  xmax=[1;0.58245800000000003]  ymin=-1  ymax=1
  removeconstantrows : neural/Processing Functions/removeconstantrows  inputSize=2  keep=[1 2]
  p : Outport  PortDimensions=2
  wires:
  mapminmax/1 -> p/1
  removeconstantrows/1 -> mapminmax/1
  fixunknowns/1 -> removeconstantrows/1
  x/1 -> fixunknowns/1

== system hyd_hyb_2_int_cont_Final_AMT/controller1/optimized controller/SOC upper 0.5/SOC upper 0.6/SOC upper 0.7/SOC upper 0.8/net_col_c_d_8_9/Process Output 1 ==
  a : Inport  PortDimensions=1
  mapminmax_reverse : neural/Processing Functions/mapminmax_reverse  xmin=0  xmax=1  ymin=-1  ymax=1
  removeconstantrows_reverse : neural/Processing Functions/removeconstantrows_reverse  inputSize=1  constants=zeros(0,1)  rearrange=1
  y : Outport  PortDimensions=1
  wires:
  removeconstantrows_reverse/1 -> y/1
  mapminmax_reverse/1 -> removeconstantrows_reverse/1
  a/1 -> mapminmax_reverse/1

== system hyd_hyb_2_int_cont_Final_AMT/controller1/optimized controller/SOC upper 0.5/SOC upper 0.6/SOC upper 0.7/SOC upper 0.8/net_col_e_f_8_9/Layer 1 ==
  "p{1}" : Inport  PortDimensions=2
  Delays 1 : Subsystem
  "IW{1,1}" : Subsystem
  "b{1}" : Constant  Value=[9.4015860759943966;-8.9623532948495601;8.5480536519185701;8.1046505410424192;-7.5466355394940079;-7.2605592645199044;-6.7644609711250361;-6.40324068377633;6.0469685190620748;-5.7413104529964567;5.1004073550828455;4.7536909688907976;-4.3869298322884216;-3.7118385502056612;3.4173879876904838;-2.9642792238956539;2.5109440040112929;2.1436189865847459;-1.7054760294924085;1.2789285491357323;0.84702857546792387;-0.42845582688182682;0.054882353957567492;-0.40580987731936785;0.83189682774366758;-1.3323426667166121;1.7017266340694932;2.2140395237166892;-2.4800599409674757;2.8411443376504515;-3.3611018732833946;-3.9122774496765476;-4.2725122406999256;4.2536055601757869;5.1225152835425725;-5.5373788998665079;5.9765064965422576;-6.4270271409881659;-6.791830750517736;-7.3042677014218906;-7.6961747552868962;8.0679800328071796;-8.5403581573270912;-8.9645856768191319;9.3914854194720938]
  netsum : Sum  Inputs=2  SaturateOnIntegerOverflow=on  InputSameDT=on  OutDataTypeStr=Inherit: Same as first input
  tansig : neural/Transfer Functions/tansig
  "a{1}" : Outport  InitialOutput=[0;0;0;0;0;0;0;0;0;0;0;0;0;0;0;0;0;0;0;0;0;0;0;0;0;0;0;0;0;0;0;0;0;0;0;0;0;0;0;0;0;0;0;0;0]
  wires:
  tansig/1 -> "a{1}"/1
  netsum/1 -> tansig/1
  "b{1}"/1 -> netsum/2
  "IW{1,1}"/1("iz{1,1}") -> netsum/1
  Delays 1/1("pd{1,1}") -> "IW{1,1}"/1("pd{1,1}")
  "p{1}"/1 -> Delays 1/1("p{1}")

== system hyd_hyb_2_int_cont_Final_AMT/controller1/optimized controller/SOC upper 0.5/SOC upper 0.6/SOC upper 0.7/SOC upper 0.8/net_col_e_f_8_9/Layer 2 ==
  "a{1} " : Inport  PortDimensions=45
  Delays 1 : Subsystem
  "LW{2,1}" : Subsystem
  "b{2}" : Constant  Value=[1.5253321238047128;1.4426726863252606;-1.3964076148505893;-1.3434292293770562;1.2678530519528122;1.1669163880968327;-1.1241349942514887;-1.0917726034495538;-1.0179705297074282;-0.95676753272242343;0.880004094253938;0.82779411887496857;0.77361446766304676;-0.70961133316188985;0.67547417475024096;0.59353382732856175;0.52119438118217298;0.42939358344025758;-0.40583901134992156;-0.33670536350227231;-0.30812213039158887;0.21614184544915765;-0.15827865619741779;0.052978289767213006;-0.0318222212966148;0.030995499762107467;0.089872985526170221;0.170835823291382;-0.23422224909781603;0.3147508551030011;-0.39562127859636015;0.4016708983328201;-0.46047284059491694;-0.51954829349618004;0.58569212638724233;0.65270315684131097;-0.67454354069254074;0.80243169197463704;0.85133965435293057;0.8963147932673079;-0.96395548478725546;-1.0113939551973554;1.108860035215596;1.084747261067099;1.2150548435091166;-1.2765324018453701;-1.3515968421724327;-1.3804162913221047;1.4444549438943957;1.5249712838830871]
  netsum : Sum  Inputs=2  SaturateOnIntegerOverflow=on  InputSameDT=on  OutDataTypeStr=Inherit: Same as first input
  tansig : neural/Transfer Functions/tansig
  "a{2}" : Outport  InitialOutput=[0;0;0;0;0;0;0;0;0;0;0;0;0;0;0;0;0;0;0;0;0;0;0;0;0;0;0;0;0;0;0;0;0;0;0;0;0;0;0;0;0;0;0;0;0;0;0;0;0;0]
  wires:
  tansig/1 -> "a{2}"/1
  netsum/1 -> tansig/1
  "b{2}"/1 -> netsum/2
  "LW{2,1}"/1("lz{2,1}") -> netsum/1
  Delays 1/1("pd{2,1}") -> "LW{2,1}"/1("ad{2,1}")
  "a{1} "/1 -> Delays 1/1("p{2}")

== system hyd_hyb_2_int_cont_Final_AMT/controller1/optimized controller/SOC upper 0.5/SOC upper 0.6/SOC upper 0.7/SOC upper 0.8/net_col_e_f_8_9/Layer 3 ==
  "a{2} " : Inport  PortDimensions=50
  Delays 1 : Subsystem
  "LW{3,2}" : Subsystem
  "b{3}" : Constant  Value=-0.73453859105110131
  netsum : Sum  Inputs=2  SaturateOnIntegerOverflow=on  InputSameDT=on  OutDataTypeStr=Inherit: Same as first input
  purelin : neural/Transfer Functions/purelin
  "a{3}" : Outport  InitialOutput=0
  wires:
  purelin/1 -> "a{3}"/1
  netsum/1 -> purelin/1
  "b{3}"/1 -> netsum/2
  "LW{3,2}"/1("lz{3,2}") -> netsum/1
  Delays 1/1("pd{3,2}") -> "LW{3,2}"/1("ad{3,2}")
  "a{2} "/1 -> Delays 1/1("p{3}")

== system hyd_hyb_2_int_cont_Final_AMT/controller1/optimized controller/SOC upper 0.5/SOC upper 0.6/SOC upper 0.7/SOC upper 0.8/net_col_e_f_8_9/Process Input 1 ==
  x : Inport  PortDimensions=2
  fixunknowns : neural/Processing Functions/fixunknowns  inputSize=2  indices=[1 2]
  mapminmax : neural/Processing Functions/mapminmax  xmin=[0.012187384778861551;0.026488162500000002]  xmax=[1.009090909090909;0.54223299999999997]  ymin=-1  ymax=1
  removeconstantrows : neural/Processing Functions/removeconstantrows  inputSize=2  keep=[1 2]
  p : Outport  PortDimensions=2
  wires:
  mapminmax/1 -> p/1
  removeconstantrows/1 -> mapminmax/1
  fixunknowns/1 -> removeconstantrows/1
  x/1 -> fixunknowns/1

== system hyd_hyb_2_int_cont_Final_AMT/controller1/optimized controller/SOC upper 0.5/SOC upper 0.6/SOC upper 0.7/SOC upper 0.8/net_col_e_f_8_9/Process Output 1 ==
  a : Inport  PortDimensions=1
  mapminmax_reverse : neural/Processing Functions/mapminmax_reverse  xmin=0  xmax=1  ymin=-1  ymax=1
  removeconstantrows_reverse : neural/Processing Functions/removeconstantrows_reverse  inputSize=1  constants=zeros(0,1)  rearrange=1
  y : Outport  PortDimensions=1
  wires:
  removeconstantrows_reverse/1 -> y/1
  mapminmax_reverse/1 -> removeconstantrows_reverse/1
  a/1 -> mapminmax_reverse/1

== system hyd_hyb_2_int_cont_Final_AMT/controller1/optimized controller/SOC upper 0.5/SOC upper 0.6/SOC upper 0.7/SOC upper 0.8/net_loc_rod_8_9/Layer 1 ==
  "p{1}" : Inport  PortDimensions=2
  Delays 1 : Subsystem
  "IW{1,1}" : Subsystem
  "b{1}" : Constant  Value=[6.9957007495819052;-6.4222898500365853;-5.788068254476527;4.9484038597923208;-4.897680334949869;4.0902305007500548;-3.4579527463580804;-2.7707675590821905;2.2287546877108686;-1.770011467044045;-1.1837111909482061;-0.033766395640138086;-0.010074994472143614;-0.76903616379233108;1.1855446863873538;1.7401032750561261;2.4956626318889397;2.9273420606852465;-3.5487048822941847;-3.9918574108068756;-4.3619449722476942;5.2498961119747447;-5.6249161050042025;6.4634990534294996;6.9541097039616186]
  netsum : Sum  Inputs=2  SaturateOnIntegerOverflow=on  InputSameDT=on  OutDataTypeStr=Inherit: Same as first input
  tansig : neural/Transfer Functions/tansig
  "a{1}" : Outport  InitialOutput=[0;0;0;0;0;0;0;0;0;0;0;0;0;0;0;0;0;0;0;0;0;0;0;0;0]
  wires:
  tansig/1 -> "a{1}"/1
  netsum/1 -> tansig/1
  "b{1}"/1 -> netsum/2
  "IW{1,1}"/1("iz{1,1}") -> netsum/1
  Delays 1/1("pd{1,1}") -> "IW{1,1}"/1("pd{1,1}")
  "p{1}"/1 -> Delays 1/1("p{1}")

== system hyd_hyb_2_int_cont_Final_AMT/controller1/optimized controller/SOC upper 0.5/SOC upper 0.6/SOC upper 0.7/SOC upper 0.8/net_loc_rod_8_9/Layer 2 ==
  "a{1} " : Inport  PortDimensions=25
  Delays 1 : Subsystem
  "LW{2,1}" : Subsystem
  "b{2}" : Constant  Value=[3.285738559317775;-3.0376074370088557;2.9182454057119536;2.7178352616345638;-2.4587927074579339;-2.4627649650599852;2.3023381037248565;2.1198885946639727;1.8964367137641158;-1.753810639868139;-1.6118339248574409;1.3623437270724821;1.2373583426900003;-1.0632509377280692;-0.90198498135918437;0.67954961164333982;-0.5916625396957329;0.40151715963968393;-0.23710697987107432;-0.071612115359177123;0.075573455100869436;0.40143850902934336;-0.44244857979555025;0.62956101630163486;-0.84379745562729247;0.930371454762837;1.0544918286478617;-1.2521280663986976;-1.4156333554037395;1.6888851421925526;1.7902496208770324;1.8134257231185751;2.0827105343371075;2.1933961234539705;2.396103863349476;-2.5699002322762587;2.7438573592567939;-2.8511956238965812;-3.1183797845775474;3.2566514179964514]
  logsig : neural/Transfer Functions/logsig
  netsum : Sum  Inputs=2  SaturateOnIntegerOverflow=on  InputSameDT=on  OutDataTypeStr=Inherit: Same as first input
  "a{2}" : Outport  InitialOutput=[0;0;0;0;0;0;0;0;0;0;0;0;0;0;0;0;0;0;0;0;0;0;0;0;0;0;0;0;0;0;0;0;0;0;0;0;0;0;0;0]
  wires:
  logsig/1 -> "a{2}"/1
  netsum/1 -> logsig/1
  "b{2}"/1 -> netsum/2
  "LW{2,1}"/1("lz{2,1}") -> netsum/1
  Delays 1/1("pd{2,1}") -> "LW{2,1}"/1("ad{2,1}")
  "a{1} "/1 -> Delays 1/1("p{2}")

== system hyd_hyb_2_int_cont_Final_AMT/controller1/optimized controller/SOC upper 0.5/SOC upper 0.6/SOC upper 0.7/SOC upper 0.8/net_loc_rod_8_9/Layer 3 ==
  "a{2} " : Inport  PortDimensions=40
  Delays 1 : Subsystem
  "LW{3,2}" : Subsystem
  "b{3}" : Constant  Value=-0.83145624638764304
  netsum : Sum  Inputs=2  SaturateOnIntegerOverflow=on  InputSameDT=on  OutDataTypeStr=Inherit: Same as first input
  purelin : neural/Transfer Functions/purelin
  "a{3}" : Outport  InitialOutput=0
  wires:
  purelin/1 -> "a{3}"/1
  netsum/1 -> purelin/1
  "b{3}"/1 -> netsum/2
  "LW{3,2}"/1("lz{3,2}") -> netsum/1
  Delays 1/1("pd{3,2}") -> "LW{3,2}"/1("ad{3,2}")
  "a{2} "/1 -> Delays 1/1("p{3}")

== system hyd_hyb_2_int_cont_Final_AMT/controller1/optimized controller/SOC upper 0.5/SOC upper 0.6/SOC upper 0.7/SOC upper 0.8/net_loc_rod_8_9/Process Input 1 ==
  x : Inport  PortDimensions=2
  fixunknowns : neural/Processing Functions/fixunknowns  inputSize=2  indices=[1 2]
  mapminmax : neural/Processing Functions/mapminmax  xmin=[0.027430680587132512;0.068007066666666671]  xmax=[0.9266183988987361;0.27192100000000002]  ymin=-1  ymax=1
  removeconstantrows : neural/Processing Functions/removeconstantrows  inputSize=2  keep=[1 2]
  p : Outport  PortDimensions=2
  wires:
  mapminmax/1 -> p/1
  removeconstantrows/1 -> mapminmax/1
  fixunknowns/1 -> removeconstantrows/1
  x/1 -> fixunknowns/1

== system hyd_hyb_2_int_cont_Final_AMT/controller1/optimized controller/SOC upper 0.5/SOC upper 0.6/SOC upper 0.7/SOC upper 0.8/net_loc_rod_8_9/Process Output 1 ==
  a : Inport  PortDimensions=1
  mapminmax_reverse : neural/Processing Functions/mapminmax_reverse  xmin=0  xmax=1  ymin=-1  ymax=1
  removeconstantrows_reverse : neural/Processing Functions/removeconstantrows_reverse  inputSize=1  constants=zeros(0,1)  rearrange=1
  y : Outport  PortDimensions=1
  wires:
  removeconstantrows_reverse/1 -> y/1
  mapminmax_reverse/1 -> removeconstantrows_reverse/1
  a/1 -> mapminmax_reverse/1

== system hyd_hyb_2_int_cont_Final_AMT/controller1/optimized controller/SOC upper 0.5/SOC upper 0.6/SOC upper 0.7/SOC under 0.8/net_col_a_b_7_8/Layer 1/Delays 1 ==
  "p{1}" : Inport  PortDimensions=2
  mux : Mux  Inputs=1
  "pd{1,1}" : Outport
  wires:
  mux/1 -> "pd{1,1}"/1
  "p{1}"/1 -> mux/1

== system hyd_hyb_2_int_cont_Final_AMT/controller1/optimized controller/SOC upper 0.5/SOC upper 0.6/SOC upper 0.7/SOC under 0.8/net_col_a_b_7_8/Layer 1/IW{1,1} ==
  "pd{1,1}" : Inport  PortDimensions=2
  "IW{1,1}(1,:)'" : Constant  Value=[-0.35647617377997598;-8.2676460038330681]
  "IW{1,1}(10,:)'" : Constant  Value=[8.1724618466293393;-1.4090893800281323]
  "IW{1,1}(11,:)'" : Constant  Value=[-5.6583295065627093;6.0581953692483541]
  "IW{1,1}(12,:)'" : Constant  Value=[-4.2662440455644184;-7.1152693972113497]
  "IW{1,1}(13,:)'" : Constant  Value=[8.031358630017758;2.0162561840220161]
  "IW{1,1}(14,:)'" : Constant  Value=[-5.3278900499296187;6.4094099373443356]
  "IW{1,1}(15,:)'" : Constant  Value=[-7.131985977957183;-4.1813157767983427]
  "IW{1,1}(16,:)'" : Constant  Value=[-0.93905683739275025;-8.2304695059797197]
  "IW{1,1}(17,:)'" : Constant  Value=[-7.3715276479010852;3.7921931410243714]
  "IW{1,1}(18,:)'" : Constant  Value=[8.2416127802679551;0.84110719468980011]
  "IW{1,1}(19,:)'" : Constant  Value=[7.1931619626456555;-4.0857855515931893]
  "IW{1,1}(2,:)'" : Constant  Value=[5.2266810116382638;6.4039586204981598]
  "IW{1,1}(20,:)'" : Constant  Value=[-8.1994640763424886;1.0931790920404731]
  "IW{1,1}(21,:)'" : Constant  Value=[6.4555426726151541;5.0566530363936328]
  "IW{1,1}(22,:)'" : Constant  Value=[8.1612750844471282;1.4182889884321903]
  "IW{1,1}(23,:)'" : Constant  Value=[8.2910343362530057;-0.77417265353998876]
  "IW{1,1}(24,:)'" : Constant  Value=[5.5645392630726578;-6.1672930029823192]
  "IW{1,1}(25,:)'" : Constant  Value=[-8.3084419032165666;-1.3187727996424765]
  "IW{1,1}(26,:)'" : Constant  Value=[7.2580127071348528;-3.9461696475692225]
  "IW{1,1}(27,:)'" : Constant  Value=[-7.381033270234461;3.6815714843334821]
  "IW{1,1}(28,:)'" : Constant  Value=[-7.5786870452751973;3.3450357137489712]
  "IW{1,1}(29,:)'" : Constant  Value=[8.0690153799601543;-1.9100893093584328]
  "IW{1,1}(3,:)'" : Constant  Value=[4.4324663496163215;-6.9671847199778201]
  "IW{1,1}(30,:)'" : Constant  Value=[-8.253479779737134;-0.3489779236507432]
  "IW{1,1}(31,:)'" : Constant  Value=[-8.1587597179163396;0.82791568295957074]
  "IW{1,1}(32,:)'" : Constant  Value=[-1.9838390141314362;-8.1837806901331707]
  "IW{1,1}(33,:)'" : Constant  Value=[-5.6562528344145333;-6.1081302358382725]
  "IW{1,1}(34,:)'" : Constant  Value=[8.2334908628753283;0.93874106230665788]
  "IW{1,1}(35,:)'" : Constant  Value=[-5.9948697585509132;5.7235516352416962]
  "IW{1,1}(4,:)'" : Constant  Value=[1.9601079068283775;8.0427372204594096]
  "IW{1,1}(5,:)'" : Constant  Value=[-5.8474920815752034;5.8752837939179772]
  "IW{1,1}(6,:)'" : Constant  Value=[-7.5317289070331332;-3.5302043552301092]
  "IW{1,1}(7,:)'" : Constant  Value=[-7.9607402696488458;2.384982730707693]
  "IW{1,1}(8,:)'" : Constant  Value=[-6.0259628008717856;-5.6504364948740786]
  "IW{1,1}(9,:)'" : Constant  Value=[5.8850098810440672;-5.8388574195215055]
  Mux : Mux  Inputs=35
  dotprod{1..35} (35 alike) : neural/Weight Functions/dotprod
  "iz{1,1}" : Outport
  wires:
  Mux/1 -> "iz{1,1}"/1
  dotprod35/1 -> Mux/35
  "IW{1,1}(35,:)'"/1 -> dotprod35/1
  dotprod34/1 -> Mux/34
  "IW{1,1}(34,:)'"/1 -> dotprod34/1
  dotprod33/1 -> Mux/33
  "IW{1,1}(33,:)'"/1 -> dotprod33/1
  dotprod32/1 -> Mux/32
  "IW{1,1}(32,:)'"/1 -> dotprod32/1
  dotprod31/1 -> Mux/31
  "IW{1,1}(31,:)'"/1 -> dotprod31/1
  dotprod30/1 -> Mux/30
  "IW{1,1}(30,:)'"/1 -> dotprod30/1
  dotprod29/1 -> Mux/29
  "IW{1,1}(29,:)'"/1 -> dotprod29/1
  dotprod28/1 -> Mux/28
  "IW{1,1}(28,:)'"/1 -> dotprod28/1
  dotprod27/1 -> Mux/27
  "IW{1,1}(27,:)'"/1 -> dotprod27/1
  dotprod26/1 -> Mux/26
  "IW{1,1}(26,:)'"/1 -> dotprod26/1
  dotprod25/1 -> Mux/25
  "IW{1,1}(25,:)'"/1 -> dotprod25/1
  dotprod24/1 -> Mux/24
  "IW{1,1}(24,:)'"/1 -> dotprod24/1
  dotprod23/1 -> Mux/23
  "IW{1,1}(23,:)'"/1 -> dotprod23/1
  dotprod22/1 -> Mux/22
  "IW{1,1}(22,:)'"/1 -> dotprod22/1
  dotprod21/1 -> Mux/21
  "IW{1,1}(21,:)'"/1 -> dotprod21/1
  dotprod20/1 -> Mux/20
  "IW{1,1}(20,:)'"/1 -> dotprod20/1
  dotprod19/1 -> Mux/19
  "IW{1,1}(19,:)'"/1 -> dotprod19/1
  dotprod18/1 -> Mux/18
  "IW{1,1}(18,:)'"/1 -> dotprod18/1
  dotprod17/1 -> Mux/17
  "IW{1,1}(17,:)'"/1 -> dotprod17/1
  dotprod16/1 -> Mux/16
  "IW{1,1}(16,:)'"/1 -> dotprod16/1
  dotprod15/1 -> Mux/15
  "IW{1,1}(15,:)'"/1 -> dotprod15/1
  dotprod14/1 -> Mux/14
  "IW{1,1}(14,:)'"/1 -> dotprod14/1
  dotprod13/1 -> Mux/13
  "IW{1,1}(13,:)'"/1 -> dotprod13/1
  dotprod12/1 -> Mux/12
  "IW{1,1}(12,:)'"/1 -> dotprod12/1
  dotprod11/1 -> Mux/11
  "IW{1,1}(11,:)'"/1 -> dotprod11/1
  dotprod10/1 -> Mux/10
  "IW{1,1}(10,:)'"/1 -> dotprod10/1
  dotprod9/1 -> Mux/9
  "IW{1,1}(9,:)'"/1 -> dotprod9/1
  dotprod8/1 -> Mux/8
  "IW{1,1}(8,:)'"/1 -> dotprod8/1
  dotprod7/1 -> Mux/7
  "IW{1,1}(7,:)'"/1 -> dotprod7/1
  dotprod6/1 -> Mux/6
  "IW{1,1}(6,:)'"/1 -> dotprod6/1
  dotprod5/1 -> Mux/5
  "IW{1,1}(5,:)'"/1 -> dotprod5/1
  dotprod4/1 -> Mux/4
  "IW{1,1}(4,:)'"/1 -> dotprod4/1
  dotprod3/1 -> Mux/3
  "IW{1,1}(3,:)'"/1 -> dotprod3/1
  dotprod2/1 -> Mux/2
  "IW{1,1}(2,:)'"/1 -> dotprod2/1
  dotprod1/1 -> Mux/1
  "pd{1,1}"/1 -> dotprod35/2, dotprod34/2, dotprod33/2, dotprod32/2, dotprod31/2, dotprod30/2, dotprod29/2, dotprod28/2, dotprod27/2, dotprod26/2, dotprod25/2, dotprod24/2, dotprod23/2, dotprod22/2, dotprod21/2, dotprod20/2, dotprod19/2, dotprod18/2, dotprod17/2, dotprod16/2, dotprod15/2, dotprod14/2, dotprod13/2, dotprod12/2, dotprod11/2, dotprod10/2, dotprod9/2, dotprod8/2, dotprod7/2, dotprod6/2, dotprod5/2, dotprod4/2, dotprod3/2, dotprod2/2, dotprod1/2
  "IW{1,1}(1,:)'"/1 -> dotprod1/1

== system hyd_hyb_2_int_cont_Final_AMT/controller1/optimized controller/SOC upper 0.5/SOC upper 0.6/SOC upper 0.7/SOC under 0.8/net_col_a_b_7_8/Layer 2/Delays 1 ==
  "p{2}" : Inport  PortDimensions=35
  mux : Mux  Inputs=1
  "pd{2,1}" : Outport
  wires:
  mux/1 -> "pd{2,1}"/1
  "p{2}"/1 -> mux/1
